simulink model "DSBSC_8"  (R2018a)
settings: Solver=VariableStepAuto  StartTime=0.0  StopTime=5.0  MaxStep=0.001  RelTol=1e-3
undefined symbols (not defined in the file or in its folder): magnitude
libraries: commanapbnd3 x3, dsparch4 x2, commchan3 x1, dspstat3 x1, commrandsrc3 x1
settings Model: Creator=sdf  LastModifiedBy=sdf

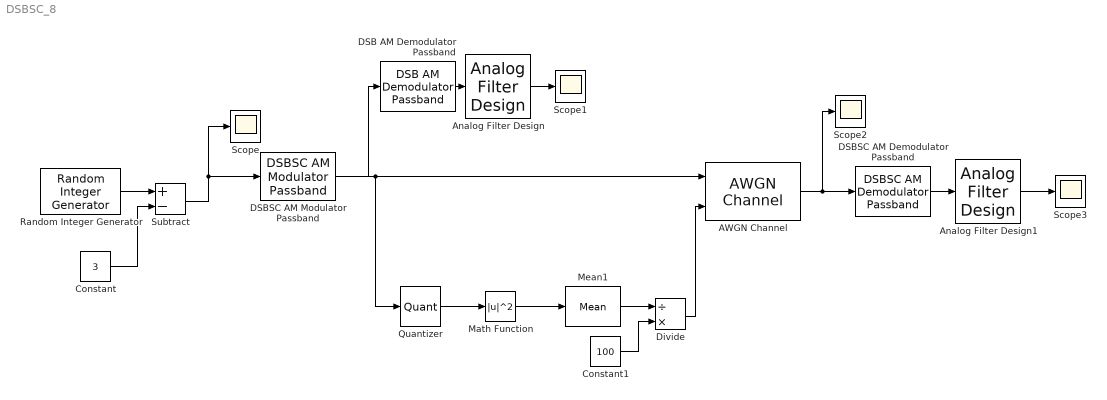
== system DSBSC_8 ==
  AWGN Channel : commchan3/AWGN Channel  InputProcessing=Columns as channels (frame based)  seed=67  noiseMode=Variance from port  EbNodB=10  EsNodB=10  SNRdB=10  bitsPerSym=1  Ps=1  Tsym=1  variance=1
  Analog Filter Design : dsparch4/Analog Filter Design  method=Butterworth  filttype=Lowpass  N=8  Wlo=30  Whi=80  Rp=2  Rs=40
  Analog Filter Design1 : dsparch4/Analog Filter Design  method=Butterworth  filttype=Lowpass  N=8  Wlo=30  Whi=80  Rp=2  Rs=40
  Constant : Constant  Value=3
  Constant1 : Constant  Value=100
  DSB AM Demodulator Passband : commanapbnd3/DSB AM Demodulator Passband  Fc=100  Ph=0  method=Butterworth  n=4  cf=300  Rp=0.1  Rs=50  Offset=4
      settings: SourceProductName=Communications System Toolbox  SourceProductBaseCode=CM
  DSBSC AM Demodulator Passband : commanapbnd3/DSBSC AM Demodulator Passband  Fc=300  Ph=0  method=Butterworth  n=4  cf=300  Rp=0.1  Rs=50
      settings: SourceProductName=Communications System Toolbox  SourceProductBaseCode=CM
  DSBSC AM Modulator Passband : commanapbnd3/DSBSC AM Modulator Passband  Fc=300  Ph=0
      settings: SourceProductName=Communications System Toolbox  SourceProductBaseCode=CM
  Divide : Product  Inputs=/*
  Math Function : Math  Operator=magnitude^2  SaturateOnIntegerOverflow=on
  Mean1 : dspstat3/Mean  run=on  InputProcessing=Columns as channels (frame based)  reset_popup=None  directionMode=Each column  dimension=1  roiEnable=off  roiType=Rectangles  roiPortion=Entire ROI  roiOutput=Individual statistics for each ROI  roiFlag=off  roundingMode=Floor  overflowMode=off  outputDataTypeStr=Inherit: Same as accumulator  outputMin=[]  outputMax=[]  outputLastDataTypeStr=Inherit: Same as accumulator
  Quantizer : Quantizer  QuantizationInterval=0.001  LinearizeAsGain=off
  Random Integer Generator : commrandsrc3/Random Integer Generator  SetSize=7  SeedSource=Parameter  Seed=1234  SampleTime=1/2  SamplesPerFrame=10  OutputDataType=double  SimulateUsing=Interpreted execution
  Scope{,1..3} (4 alike) : Scope
  Subtract : Sum  Inputs=+-
  wires:
  Random Integer Generator/1 -> Subtract/1
  Constant/1 -> Subtract/2
  Subtract/1 -> DSBSC AM Modulator Passband/1, Scope/1
  DSBSC AM Modulator Passband/1 -> AWGN Channel/1, DSB AM Demodulator Passband/1, Quantizer/1
  Quantizer/1 -> Math Function/1
  Math Function/1 -> Mean1/1
  Mean1/1 -> Divide/1
  DSB AM Demodulator Passband/1 -> Analog Filter Design/1
  Analog Filter Design/1 -> Scope1/1
  Constant1/1 -> Divide/2
  Divide/1 -> AWGN Channel/2
  AWGN Channel/1 -> DSBSC AM Demodulator Passband/1, Scope2/1
  DSBSC AM Demodulator Passband/1 -> Analog Filter Design1/1
  Analog Filter Design1/1 -> Scope3/1
